simulink model "equlibrium"  (R2018a)
settings: Solver=ode3  StartTime=0.0  StopTime=5  FixedStep=0.01  RelTol=1e-3  EnableMultiTasking=on
values from neighbouring files (symbols this model uses):
  A = [0,1; g/l,0]    [in.m]
  b = [0;-1/m/l/l]    [in.m]
  c = [1,0;0,1]    [in.m]
  cn = [1,0;0,0]    [in.m]
  k = (place(A,b,p))    [in.m]
  l = (place(A',cn',p))'    [in.m]
  th0 = 5    [in.m]
  v0 = 3    [in.m]
settings Model: Creator=Admin  LastModifiedBy=cooks
settings DataIOCC: LimitDataPoints=on  SaveFormat=Array  SignalLoggingSaveFormat=ModelDataLogs
settings OptimizationCC: ExpressionDepthLimit=2147483647  LifeSpan=inf
settings DebuggingCC: UnderspecifiedInitializationDetection=Classic  MergeDetectMultiDrivingBlocksExec=none  SolverPrmCheckMsg=warning  FcnCallInpInsideContextMsg=warning  StateNameClashWarn=warning  SFUnexpectedBacktrackingDiag=warning  SFNoUnconditionalDefaultTransitionDiag=warning  SFExecutionAtInitializationDiag=none
settings HardwareCC: ProdBitPerPointer=32  ProdBitPerSizeT=32  ProdBitPerPtrDiffT=32  ProdLargestAtomicFloat=None  ProdIntDivRoundTo=Undefined  ProdEndianess=Unspecified  ProdWordSize=32  ProdHWDeviceType=32-bit Generic
settings ModelReferenceCC: PropagateSignalLabelsOutOfModel=off
settings CodeAppCC: StateflowObjectComments=on
settings GRTTargetCC: TargetLangStandard=C89/C90 (ANSI)  GeneratePreprocessorConditionals=Disable all  CombineOutputUpdateFcns=off  GRTInterface=on
settings ConfigComp: CovMetricSettings=dw  CovHtmlReporting=on  CovSaveCumulativeToWorkspaceVar=on  CovSaveSingleToWorkspaceVar=on  CovExternalEMLEnable=off

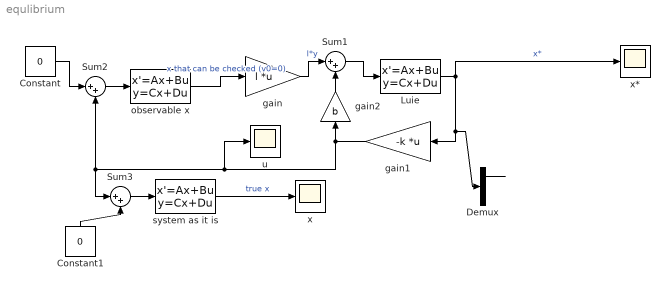
== system equlibrium ==
  Constant : Constant  Value=0
  Constant1 : Constant  Value=0
  Demux : Demux  Outputs=2
  Luie : StateSpace  A=A-l*c  B=eye(2)  C=eye(2)  D=zeros(2)  InitialCondition=[th0 0]
  Sum1 : Sum  Inputs=|++
  Sum2 : Sum  Inputs=|++
  Sum3 : Sum  Inputs=|++
  gain : Gain  Gain=l  Multiplication=Matrix(K*u) (u vector)
  gain1 : Gain  Gain=-k  Multiplication=Matrix(K*u) (u vector)
  gain2 : Gain  Gain=b
  observable x : StateSpace  A=A  B=b  C=cn  D=[0;0]  InitialCondition=[th0 v0]
  system as it is : StateSpace  A=A  B=b  C=[1,0;0,1]  D=[0;0]  InitialCondition=[th0 v0]
  u : Scope
  x : Scope
  x* : Scope
  wires:
  system as it is/1 -> x/1  "true x"
  Luie/1 -> x*/1, gain1/1, Demux/1  "x*"
  Sum1/1 -> Luie/1
  observable x/1 -> gain/1  "x that can be checked (v0=0)"
  gain/1 -> Sum1/1  "l*y"
  Sum2/1 -> observable x/1
  Sum3/1 -> system as it is/1
  gain1/1 -> u/1, Sum2/2, Sum3/1, gain2/1
  gain2/1 -> Sum1/2
  Constant/1 -> Sum2/1
  Constant1/1 -> Sum3/2
  Demux/1 -> ?
